simulink library "tetherDragForce_ul"  (R2018b)
settings: Solver=VariableStepAuto  StartTime=0.0  StopTime=10.0  RelTol=1e-3
values from neighbouring files (symbols this model uses):
  Cd = 0.5    [tetherDragForce_ts.m]
  D = NaN(6*(N-2),1)    [tether_ode.m]
  dia_t = 0.01    [tetherDragForce_ts.m]
  N = 5    [tetherDragForce_ts.m]    (also in tether_ode.m = sz(1))
  rho_fluid = 1000    [tetherDragForce_ts.m]
settings Model: Creator=asiddiq2  LastModifiedBy=mcobb

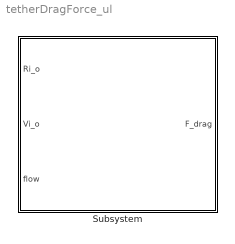
== system tetherDragForce_ul ==
  Subsystem : Subsystem  mask{Cd=Cd, rho_fluid=rho_fluid, dia_t=dia_t}
      mask prompts: Cd "Drag coefficient"; rho_fluid "Fluid density (kg/m^3)"; dia_t "Tether diameter (m)"

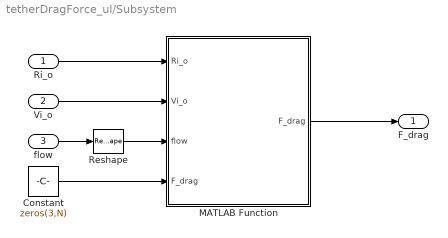
== system tetherDragForce_ul/Subsystem ==
  Ri_o : Inport
  Vi_o : Inport  Port=2
  flow : Inport  Port=3
  Constant : Constant  Value=zeros(3,N)
  MATLAB Function : MATLAB Function  TreatAsAtomicUnit=on
  Reshape : Reshape  OutputDimensionality=Column vector (2-D)
  F_drag : Outport
  wires:
  Ri_o/1 -> MATLAB Function/1(Ri_o)
  Vi_o/1 -> MATLAB Function/2(Vi_o)
  Constant/1 -> MATLAB Function/4("F_drag ")
  MATLAB Function/1(F_drag) -> F_drag/1
  flow/1 -> Reshape/1
  Reshape/1 -> MATLAB Function/3(flow)

== matlab function tetherDragForce_ul/Subsystem/MATLAB Function ==
  data: Ri_o input; F_drag output; Vi_o input; flow input; F_drag input; Cd parameter; dia_t parameter; rho_fluid parameter; N parameter
function F_drag = fcn(Ri_o,Vi_o,flow,F_drag,Cd, dia_t, rho_fluid, N)

Ve = zeros(3,N-1);
Vrel = zeros(3,N-1);
drag_direction = zeros(3,N-1);
drag = zeros(3,N-1);

qe = zeros(N-1,1);
di = zeros(N-1,1);
th = zeros(N-1,1);
S = zeros(N-1,1);

% elemental velocity
for i = 1:N-1
    
    % relative velocity
    Ve(:,i) = (Vi_o(:,i) + Vi_o(:,i+1))/2;
    Vrel(:,i) = flow - Ve(:,i);
    Vrel(3,i) = 0;
    % drag direction
    if norm(Vrel(:,i)) > 1e-3
        drag_direction(:,i) = Vrel(:,i)/norm(Vrel(:,i));
    else
        drag_direction(:,i) = zeros(3,1);
    end
    
    % dynamic pressure
    qe(i) = 0.5*rho_fluid*norm(Vrel(:,i))^2;
    
    % projected area
    di(i) = norm(Ri_o(:,i+1)-Ri_o(:,i));
    th(i) = atan( (Ri_o(3,i+1)-Ri_o(3,i))/norm(Ri_o(1:2,i+1)-Ri_o(1:2,i)) );
    S(i) = di(i)*dia_t*sin(th(i));
    
    drag(:,i) = 0.5*rho_fluid*Cd*Vrel(:,i)*norm(Vrel(:,i))*S(i);
    x=1;
end

% drag force acting on each node'
for i = 1:N
    if i == 1
        F_drag(:,i) = drag(:,i)/2;
    elseif i> 1 && i < N
        F_drag(:,i) = (drag(:,i-1) + drag(:,i))/2;
    elseif i == N
        F_drag(:,i) = drag(:,i-1)/2;
    end
end

end
